simulink model "arduSon"  (R2021b)
settings: Solver=FixedStepAuto  StartTime=0.0  StopTime=5000  RelTol=1e-3
model workspace (MAT data in the model file):
  constantVal = 22
libraries: arduinolib x2
settings Model: ExtModeTrigDuration=2  Creator=OmerFarukCanbaz  LastModifiedBy=OmerFarukCanbaz
settings OptimizationCC: EnhancedBackFolding=on  PassReuseOutputArgsAs=Individual arguments  ZeroExternalMemoryAtStartup=off  ZeroInternalMemoryAtStartup=off  MaxStackSize=64  OptimizeBlockOrder=speed  DifferentSizesBufferReuse=on  OptimizationCustomize=off  EfficientTunableParamExpr=on
settings DebuggingCC: ParameterTunabilityLossMsg=error
settings HardwareCC: ProdBitPerInt=16  ProdBitPerPointer=16  ProdBitPerSizeT=16  ProdBitPerPtrDiffT=16  ProdLargestAtomicFloat=None  ProdWordSize=8  ProdHWDeviceType=Atmel->AVR  UseEmbeddedCoderFeatures=off
settings SFSimCC: MATLABDynamicMemAlloc=off
settings RTWCC: Description=Embedded Coder  SystemTargetFile=ert.tlc  HardwareBoard=Arduino Uno  TemplateMakefile=ert_default_tmf  Toolchain=Arduino AVR
settings CodeAppCC: ForceParamTrailComments=on  IgnoreCustomStorageClasses=off  OperatorAnnotations=on  SimulinkDataObjDesc=on  SFDataObjDesc=on  InsertBlockDesc=on
settings ERTTargetCC: SupportContinuousTime=on  SupportNonInlinedSFcns=on  SupportVariableSizeSignals=on  ExtModeTransport=3  ExtModeStaticAlloc=on  ExtModeStaticAllocSize=250  ExtModeMexFile=ext_xcp  ExtModeIntrfLevel=Level2 - Open

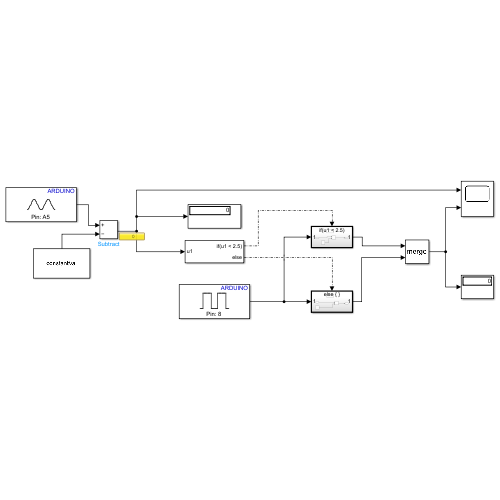
[thumbnail: Simulink's stored preview of the top-level diagram]
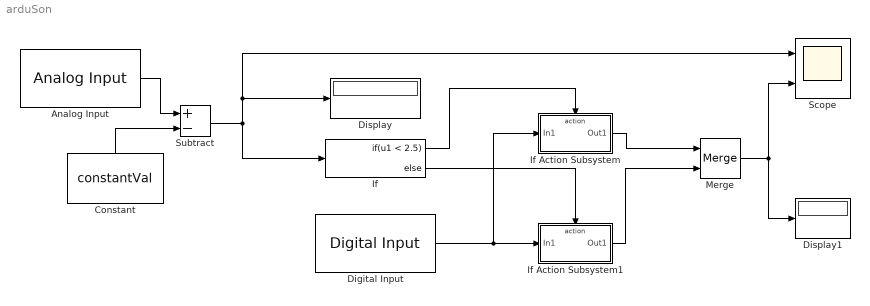
== system arduSon ==
  Analog Input : arduinolib/Analog Input  pinNumber=5  ReadResultsOnly=off  ConversionTriggerSource=Software  ExternalTriggerType=uint32( 0 )  OutputDataType=uint16  EnableConversionCompleteNotify=off  EnableOuputStatus=off  SampleTime=0.1  blockPlatform=arduino
  Constant : Constant  Value=constantVal
  Digital Input : arduinolib/Digital Input  pinNumber=8  mode=Default  Direction=input  SampleTime=0.1  blockPlatform=arduino
  Display : Display
  Display1 : Display
  If : If  IfExpression=u1 < 2.5
  If Action Subsystem : Subsystem  TreatAsAtomicUnit=on
  If Action Subsystem1 : Subsystem  TreatAsAtomicUnit=on
  Merge : Merge
  Scope : Scope  NumInputPorts=2
  Subtract : Sum  Inputs=+-
  wires:
  Subtract/1 -> Scope/1, Display/1, If/1
  Analog Input/1 -> Subtract/1
  Constant/1 -> Subtract/2
  If/2 -> If Action Subsystem1/Action
  Merge/1 -> Display1/1, Scope/2
  If Action Subsystem1/1(Out1) -> Merge/2
  If Action Subsystem/1(Out1) -> Merge/1
  If/1 -> If Action Subsystem/Action
  Digital Input/1 -> If Action Subsystem1/1(In1), If Action Subsystem/1(In1)

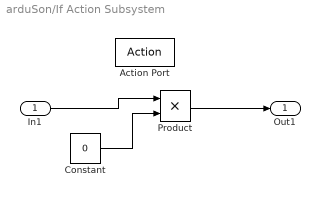
== system arduSon/If Action Subsystem ==
  In1 : Inport
  Action Port : ActionPort  ActionPortLabel=if(u1 < 2.5)
  Constant : Constant  Value=0
  Product : Product
  Out1 : Outport
  wires:
  In1/1 -> Product/1
  Constant/1 -> Product/2
  Product/1 -> Out1/1

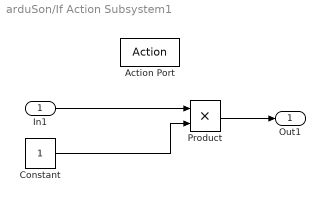
== system arduSon/If Action Subsystem1 ==
  In1 : Inport
  Action Port : ActionPort  ActionPortLabel=else
  Constant : Constant
  Product : Product
  Out1 : Outport
  wires:
  In1/1 -> Product/1
  Constant/1 -> Product/2
  Product/1 -> Out1/1
